simulink model "perro"  (R2012b)
settings: Solver=ode45  StartTime=0.0  StopTime=10.0  RelTol=1e-3
libraries: simulink x1
settings Model: Creator=Daniel  LastModifiedBy=Daniel

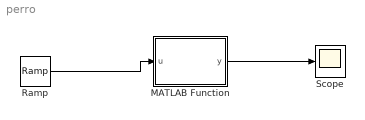
== system perro ==
  MATLAB Function : MATLAB Function  TreatAsAtomicUnit=on
  Ramp : simulink/Sources/Ramp  slope=1  start=0  X0=0
  Scope : Scope
  wires:
  Ramp/1 -> MATLAB Function/1(u)
  MATLAB Function/1(y) -> Scope/1

== matlab function perro/MATLAB Function ==
  data: u input; y output
function y = fcn(u)
%#codegen



y = sin(u)+cos(u);
